simulink model "Sim_Modell_RFJ"  (R2020b)
settings: Solver=VariableStepAuto  StartTime=0.0  StopTime=10.0  RelTol=1e-3
undefined symbols (not defined in the file or in its folder): ACD120_80_Rotor, ACD120_80_Stator, Ausleger, Auslegerplatte, DistanzhuelseGP, Federbolzen, Grundplatte, Heidenhain_ERN_1080, Lagerdeckel_oben, Lagerdeckel_unten, par_imp, par_reg, parSys, Seitenplatte, Visualisierung, Welle, X, Y, Z
libraries: sm_lib x37, fl_lib x7, nesl_utility x7, cstblocks x2, simulink x1
(part 1 of 3)
settings Model: Creator=ukn  LastModifiedBy=Simon

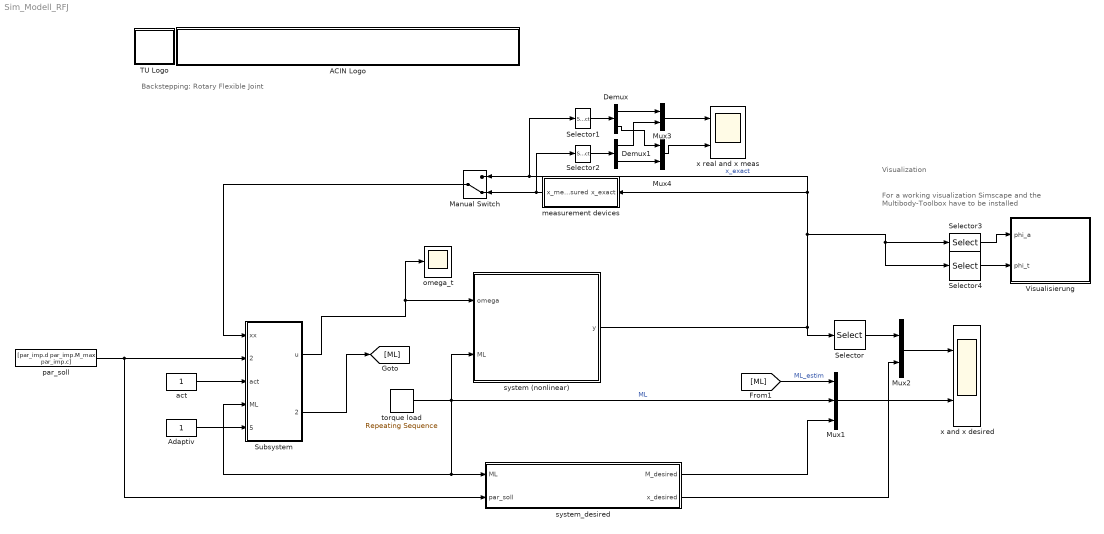
== system Sim_Modell_RFJ ==
  note: For a working visualization Simscape and
      | the Multibody-Toolbox have to be installed
  note: Backstepping: Rotary Flexible Joint
  note: Visualization
  ACIN Logo : Subsystem
      mask init:
      | s = get_param(gcb,'UserData');
      mask Display:
      | image(s.logo,[0 0 439 45]);
      | %axis image
  Adaptiv : Constant
  Demux : Demux  Outputs=2
  Demux1 : Demux  Outputs=2
  Manual Switch : ManualSwitch  CurrentSetting=0
  Mux1 : Mux  Inputs=3
  Mux2 : Mux  Inputs=2
  Mux3 : Mux  Inputs=2
  Mux4 : Mux  Inputs=2
  Selector : Selector  InputPortWidth=3  IndexOptions=Index vector (dialog)  Indices=[1 2]  OutputSizes=1
  Selector1 : Selector  InputPortWidth=3  IndexOptions=Index vector (dialog)  Indices=[1 2]  OutputSizes=1
  Selector2 : Selector  InputPortWidth=3  IndexOptions=Index vector (dialog)  Indices=[1 2]  OutputSizes=1
  Selector3 : Selector  InputPortWidth=3  IndexOptions=Index vector (dialog)  Indices=[1]  OutputSizes=1
  Selector4 : Selector  InputPortWidth=3  IndexOptions=Index vector (dialog)  Indices=[3]  OutputSizes=1
  Subsystem : Subsystem
  TU Logo : Subsystem
      mask init:
      | s = get_param(gcb,'UserData');
      mask Display: image(s.logo,[0 0 45 45]);
  Visualisierung : Subsystem
  act : Constant
  measurement devices : Subsystem
  omega_t : Scope
  par_soll : Constant  Value=[par_imp.d par_imp.M_max par_imp.c]
  system (nonlinear) : Subsystem
      mask Display: image('$imagefile'); % Use "Edit Image" on toolstrip to change.
  system_desired : Subsystem
      mask init:
      | resources = get_param(gcb,'UserData');
      mask Display:
      | image(resources.logo);
      | port_label('output', 1, 'M_desired');
      | port_label('output', 2, 'x_desired');
      | port_label('input', 1, 'ML');
      | port_label('input', 2, 'par_soll');
  torque load : simulink/Sources/Repeating Sequence  rep_seq_t=[0 0.5 1 1.5 1.50001 5]  rep_seq_y=[0 0 1 1 0 0]*0.1
  x and x desired : Scope  NumInputPorts=2
  x real and x meas : Scope  NumInputPorts=2
  wires:
  system (nonlinear)/1(y) -> Selector/1, Selector4/1, Selector3/1, measurement devices/1(x_exact), Manual Switch/1, Selector1/1  "x_exact"
  Demux1/1 -> Mux3/2
  measurement devices/1(x_measured) -> Manual Switch/2, Selector2/1
  Mux3/1 -> x real and x meas/1
  Demux/2 -> Mux4/1
  par_soll/1 -> system_desired/2(par_soll), Subsystem/2(par_soll)
  torque load/1 -> system_desired/1(ML), Subsystem/4(ML), system (nonlinear)/2(ML), Mux1/2  "ML"
  system_desired/1(M_desired) -> Mux1/3
  Mux2/1 -> x and x desired/1
  Selector1/1 -> Demux/1
  system_desired/2(x_desired) -> Mux2/2
  Mux4/1 -> x real and x meas/2
  Mux1/1 -> x and x desired/2
  Demux/1 -> Mux3/1
  [ML] -> Mux1/1  "ML_estim"
  Selector/1 -> Mux2/1
  Selector2/1 -> Demux1/1
  Demux1/2 -> Mux4/2
  Selector3/1 -> Visualisierung/1(phi_a)
  Selector4/1 -> Visualisierung/2(phi_t)
  Subsystem/1(u) -> omega_t/1, system (nonlinear)/1(omega)
  Manual Switch/1 -> Subsystem/1(xx)
  act/1 -> Subsystem/3(act)
  Subsystem/2(ML_est) -> [ML]
  Adaptiv/1 -> Subsystem/5(Adaptiv)

== system Sim_Modell_RFJ/ACIN Logo ==

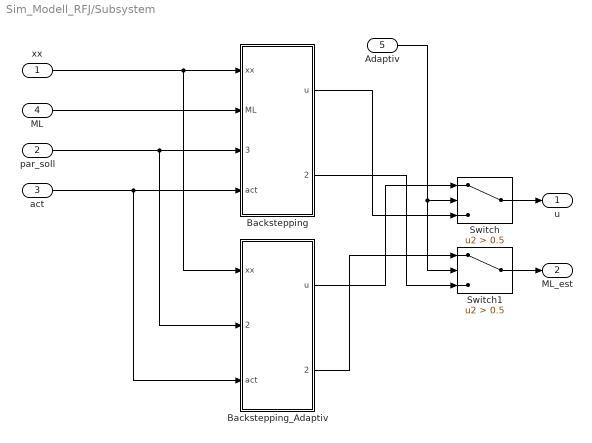
== system Sim_Modell_RFJ/Subsystem ==
  xx : Inport
  par_soll : Inport  Port=2
  act : Inport  Port=3
  ML : Inport  Port=4
  Adaptiv : Inport  Port=5
  Backstepping : MATLAB Function  TreatAsAtomicUnit=on
  Backstepping_Adaptiv : MATLAB Function  TreatAsAtomicUnit=on
  Switch : Switch  Criteria=u2 > Threshold  Threshold=0.5
  Switch1 : Switch  Criteria=u2 > Threshold  Threshold=0.5
  u : Outport
  ML_est : Outport  Port=2
  wires:
  xx/1 -> Backstepping_Adaptiv/1(xx), Backstepping/1(xx)
  ML/1 -> Backstepping/2(ML)
  par_soll/1 -> Backstepping_Adaptiv/2(par_soll), Backstepping/3(par_soll)
  act/1 -> Backstepping_Adaptiv/3(act), Backstepping/4(act)
  Switch/1 -> u/1
  Switch1/1 -> ML_est/1
  Adaptiv/1 -> Switch1/2, Switch/2
  Backstepping_Adaptiv/1(u) -> Switch/1
  Backstepping/1(u) -> Switch/3
  Backstepping_Adaptiv/2(ML_est) -> Switch1/1
  Backstepping/2(ML_est) -> Switch1/3

== system Sim_Modell_RFJ/TU Logo ==
